simulink model "MSFartoystyring_speed_1_7"  (R2018b)
settings: Solver=ode45  StartTime=tstart  StopTime=tstop  RelTol=1e-3  EnableMultiTasking=on
values from neighbouring files (symbols this model uses):
  c = 0    [find_nomoto_param.m]    (also in plotting.m; run.m)
  cutoff = 10    [run.m]
  Kd = (2*damping*wn-1)/(-K)    [run.m]
  Kd_sp = -0.2    [run.m]
  Ki_sp = 0.001    [run.m]
  Kp = wn^2*T/-K    [run.m]
  Kp_sp = -50    [run.m]
  p0 = zeros(2,1)    [find_nomoto_param.m]    (also in plotting.m; run.m = [0,0]')
  psi0 = 0    [find_nomoto_param.m]    (also in plotting.m; run.m = 1.0471975512)
  r0 = 0    [find_nomoto_param.m]    (also in plotting.m; run.m)
  tsamp = 10    [find_nomoto_param.m]    (also in plotting.m; run.m)
  v0 = [6.63 0]'    [find_nomoto_param.m]    (also in plotting.m; run.m)
undefined symbols (not defined in the file or in its folder): msfartoystyring
settings Model: ExtModeAutoUpdateStatusClock=off  Creator=christh  LastModifiedBy=dino
settings DataIOCC: LimitDataPoints=on  SaveFormat=Array  SignalLoggingSaveFormat=ModelDataLogs
settings OptimizationCC: ExpressionDepthLimit=2147483647  InitFltsAndDblsToZero=on  LifeSpan=inf
settings DebuggingCC: UnderspecifiedInitializationDetection=Classic  MergeDetectMultiDrivingBlocksExec=none  SolverPrmCheckMsg=warning  FcnCallInpInsideContextMsg=warning  StateNameClashWarn=warning  SFUnexpectedBacktrackingDiag=warning  SFNoUnconditionalDefaultTransitionDiag=warning
settings HardwareCC: ProdBitPerPointer=32  ProdBitPerSizeT=32  ProdBitPerPtrDiffT=32  ProdLargestAtomicFloat=None  ProdIntDivRoundTo=Undefined  ProdEndianess=Unspecified  ProdWordSize=32  ProdHWDeviceType=32-bit Generic
settings ModelReferenceCC: PropagateSignalLabelsOutOfModel=off
settings SFSimCC: SimUseLocalCustomCode=off
settings RTWCC: RTWUseLocalCustomCode=off
settings CodeAppCC: StateflowObjectComments=on
settings GRTTargetCC: TargetLangStandard=C89/C90 (ANSI)  GeneratePreprocessorConditionals=Disable all  CombineOutputUpdateFcns=off  GRTInterface=on
settings ConfigComp: CovMetricSettings=dw  CovHtmlReporting=on  CovSaveCumulativeToWorkspaceVar=on  CovSaveSingleToWorkspaceVar=on  CovExternalEMLEnable=off

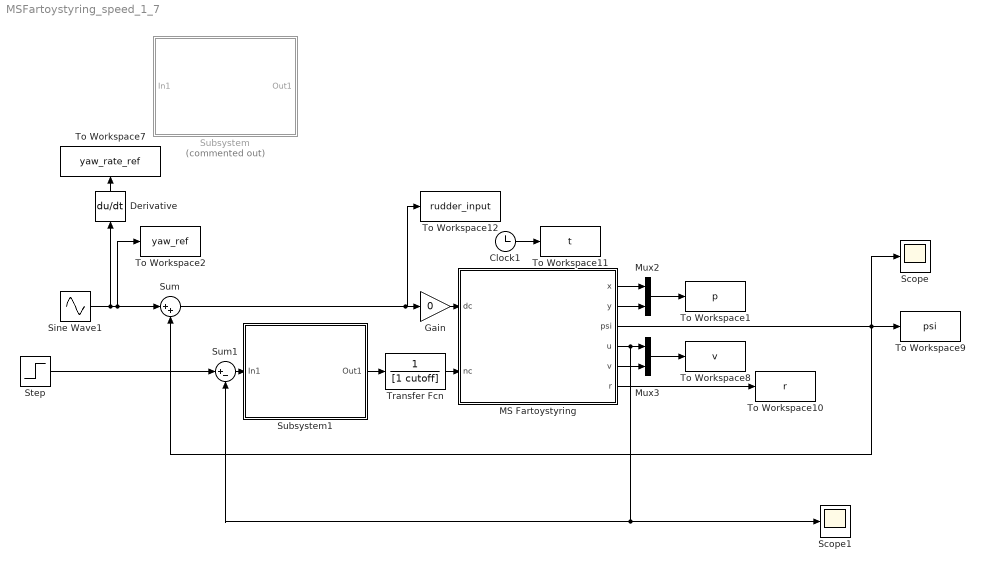
== system MSFartoystyring_speed_1_7 ==
  Clock1 : Clock
  Derivative : Derivative
  Gain : Gain  Gain=0
  MS Fartoystyring : Subsystem  mask(MS Fartoystyring for Assignment 3 G&C){x0=p0(1), y0=p0(2), u0=v0(1), v0=v0(2), psi0=psi0, r0=r0, c=c}
      mask prompts: x0 "x(t0) (m)"; y0 "y(t0) (m)"; u0 "u(t0) (m/s)"; v0 "v(t0) (m/s)"; psi0 "psi(t0) (rad)"; r0 "r(t0) (rad/s)"; c "current (0 or 1)"
      mask help:
      | Block corresponding to Figure 1 in the assignment text. Gives the response of the ship.
      |
      | The design speed of MS Fartoystyring is u=8.23 m/s.
      |
      | Input:
      | dc: commanded rudder (rad), dmax=25*pi/180
      | nc: commanded shaft speed (rad/s), nmax=85*2*pi/60
      |
      | Output:
      | x: north pos (m)
      | y: east pos (m)
      | u: surge (m/s)
      | v: sway (m/s)
      | psi: heading (rad)
      | r: yaw (rad/s)
      mask Help: Comments, bugs and help requests can be directed to the TA. Email on course website.
  Mux2 : Mux  Inputs=2
  Mux3 : Mux  Inputs=2
  Scope : Scope
  Scope1 : Scope
  Sine Wave1 : Sin  Amplitude=0.4  Frequency=0.004  SampleTime=0
  Step : Step  Time=1250*tsamp  Before=3  After=7  SampleTime=0
  Subsystem : Subsystem  Commented=on
  Subsystem1 : Subsystem
  Sum : Sum  Inputs=|++
  Sum1 : Sum  Inputs=|+-
  To Workspace1 : ToWorkspace  VariableName=p  SampleTime=tsamp
  To Workspace10 : ToWorkspace  VariableName=r  SampleTime=tsamp
  To Workspace11 : ToWorkspace  VariableName=t  SampleTime=tsamp
  To Workspace12 : ToWorkspace  VariableName=rudder_input  SampleTime=tsamp
  To Workspace2 : ToWorkspace  VariableName=yaw_ref  SampleTime=tsamp
  To Workspace7 : ToWorkspace  VariableName=yaw_rate_ref  SampleTime=tsamp
  To Workspace8 : ToWorkspace  VariableName=v  SampleTime=tsamp
  To Workspace9 : ToWorkspace  VariableName=psi  SampleTime=tsamp
  Transfer Fcn : TransferFcn  Denominator=[1 cutoff]
  wires:
  Sum/1 -> Gain/1, To Workspace12/1
  Sine Wave1/1 -> Sum/1, To Workspace2/1, Derivative/1
  MS Fartoystyring/5(v) -> Mux3/2
  MS Fartoystyring/6(r) -> To Workspace10/1
  Mux2/1 -> To Workspace1/1
  MS Fartoystyring/3(psi) -> Scope/1, Sum/2, To Workspace9/1
  Clock1/1 -> To Workspace11/1
  MS Fartoystyring/1(x) -> Mux2/1
  Mux3/1 -> To Workspace8/1
  Derivative/1 -> To Workspace7/1
  MS Fartoystyring/2(y) -> Mux2/2
  Gain/1 -> MS Fartoystyring/1(dc)
  Sum1/1 -> Subsystem1/1(In1)
  Step/1 -> Sum1/1
  MS Fartoystyring/4(u) -> Sum1/2, Scope1/1, Mux3/1
  Transfer Fcn/1 -> MS Fartoystyring/2(nc)
  Subsystem1/1(Out1) -> Transfer Fcn/1

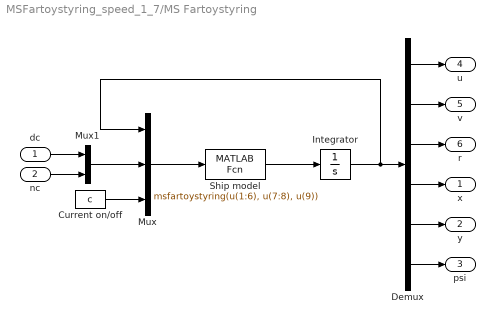
== system MSFartoystyring_speed_1_7/MS Fartoystyring ==
  dc : Inport
  nc : Inport  Port=2
  Current on/off : Constant  Value=c
  Demux : Demux  Outputs=6
  Integrator : Integrator  InitialCondition=[u0 v0 r0 x0 y0 psi0]'
  Mux : Mux  Inputs=3
  Mux1 : Mux  Inputs=2
  Ship model : MATLABFcn  MATLABFcn=msfartoystyring(u(1:6), u(7:8), u(9))  OutputDimensions=6
  x : Outport
  y : Outport  Port=2
  psi : Outport  Port=3
  u : Outport  Port=4
  v : Outport  Port=5
  r : Outport  Port=6
  wires:
  Integrator/1 -> Mux/1, Demux/1
  Mux1/1 -> Mux/2
  dc/1 -> Mux1/1
  nc/1 -> Mux1/2
  Demux/1 -> u/1
  Demux/2 -> v/1
  Demux/3 -> r/1
  Demux/4 -> x/1
  Demux/5 -> y/1
  Demux/6 -> psi/1
  Current on/off/1 -> Mux/3
  Ship model/1 -> Integrator/1
  Mux/1 -> Ship model/1

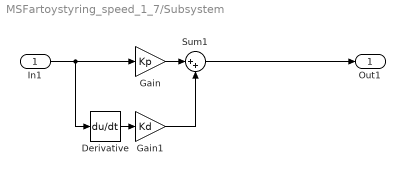
== system MSFartoystyring_speed_1_7/Subsystem ==
  In1 : Inport
  Derivative : Derivative
  Gain : Gain  Gain=Kp
  Gain1 : Gain  Gain=Kd
  Sum1 : Sum  Inputs=|++
  Out1 : Outport
  wires:
  Sum1/1 -> Out1/1
  Derivative/1 -> Gain1/1
  In1/1 -> Derivative/1, Gain/1
  Gain1/1 -> Sum1/2
  Gain/1 -> Sum1/1

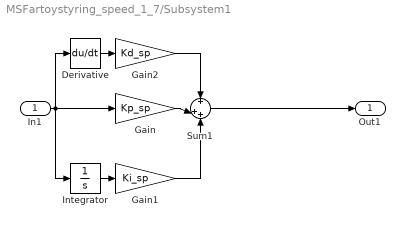
== system MSFartoystyring_speed_1_7/Subsystem1 ==
  In1 : Inport
  Derivative : Derivative
  Gain : Gain  Gain=Kp_sp
  Gain1 : Gain  Gain=Ki_sp
  Gain2 : Gain  Gain=Kd_sp
  Integrator : Integrator
  Sum1 : Sum  Inputs=+|++
  Out1 : Outport
  wires:
  Sum1/1 -> Out1/1
  In1/1 -> Derivative/1, Integrator/1, Gain/1
  Integrator/1 -> Gain1/1
  Derivative/1 -> Gain2/1
  Gain1/1 -> Sum1/3
  Gain/1 -> Sum1/2
  Gain2/1 -> Sum1/1
